simulink model "Utkarsh_2005574_R_W3_P1"  (R2021a)
settings: Solver=VariableStepAuto  StartTime=0.0  StopTime=10.0  RelTol=1e-3
settings Model: Creator=Utkarsh Anand  LastModifiedBy=Utkarsh Anand

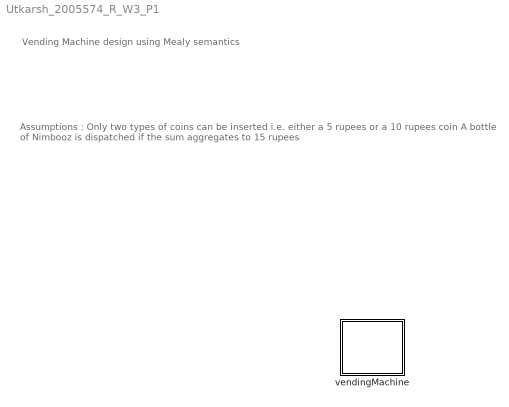
== system Utkarsh_2005574_R_W3_P1 ==
  note: Assumptions :
      | Only two types of coins can be inserted i.e. either a 5 rupees or a 10 rupees coin
      | A bottle of Nimbooz is dispatched if the sum aggregates to 15 rupees
  note: Vending Machine design using Mealy semantics
  vendingMachine : Stateflow chart  TreatAsAtomicUnit=on

== stateflow chart Utkarsh_2005574_R_W3_P1/vendingMachine ==
  state noCoinAvailable
  state gotTenRupeeCoin
  state gotFiveRupeeCoin
  (default) -> noCoinAvailable
